simulink library "limitVelocityByPositionLimits"  (R2016b)
settings: Solver=VariableStepAuto  StartTime=0.0  StopTime=10.0  RelTol=1e-3
libraries: simulink x4
settings Model: Creator=MIRACLE  LastModifiedBy=MIRACLE

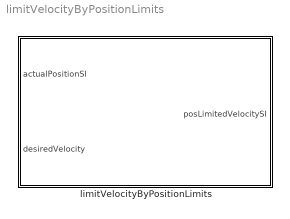
== system limitVelocityByPositionLimits ==
  limitVelocityByPositionLimits : Subsystem  mask{upperJointLimit=0, lowerJointLimit=0}

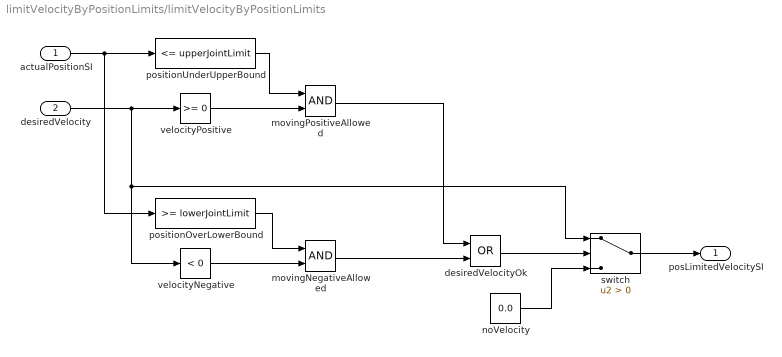
== system limitVelocityByPositionLimits/limitVelocityByPositionLimits ==
  actualPositionSI : Inport
  desiredVelocity : Inport  Port=2
  desiredVelocityOk : Logic  Operator=OR  AllPortsSameDT=off  OutDataTypeStr=boolean
  movingNegativeAllowed : Logic  AllPortsSameDT=off  OutDataTypeStr=boolean
  movingPositiveAllowed : Logic  AllPortsSameDT=off  OutDataTypeStr=boolean
  noVelocity : Constant  Value=0.0
  positionOverLowerBound : simulink/Logic and Bit Operations/Compare To Constant  relop=>=  const=lowerJointLimit  OutDataTypeStr=boolean
  positionUnderUpperBound : simulink/Logic and Bit Operations/Compare To Constant  relop=<=  const=upperJointLimit  OutDataTypeStr=boolean
  switch : Switch  Criteria=u2 > Threshold
  velocityNegative : simulink/Logic and Bit Operations/Compare To Zero  relop=<  OutDataTypeStr=boolean
  velocityPositive : simulink/Logic and Bit Operations/Compare To Zero  relop=>=  OutDataTypeStr=boolean
  posLimitedVelocitySI : Outport
  wires:
  velocityPositive/1 -> movingPositiveAllowed/2
  velocityNegative/1 -> movingNegativeAllowed/2
  positionUnderUpperBound/1 -> movingPositiveAllowed/1
  movingNegativeAllowed/1 -> desiredVelocityOk/2
  movingPositiveAllowed/1 -> desiredVelocityOk/1
  positionOverLowerBound/1 -> movingNegativeAllowed/1
  noVelocity/1 -> switch/3
  desiredVelocityOk/1 -> switch/2
  actualPositionSI/1 -> positionUnderUpperBound/1, positionOverLowerBound/1
  desiredVelocity/1 -> velocityNegative/1, switch/1, velocityPositive/1
  switch/1 -> posLimitedVelocitySI/1
